simulink model "Par8_11"  (R2018a)
settings: Solver=FixedStepAuto  StartTime=0.0  StopTime=50  FixedStep=0.01  RelTol=1e-3
settings Model: Creator=wangluo  LastModifiedBy=wangluo

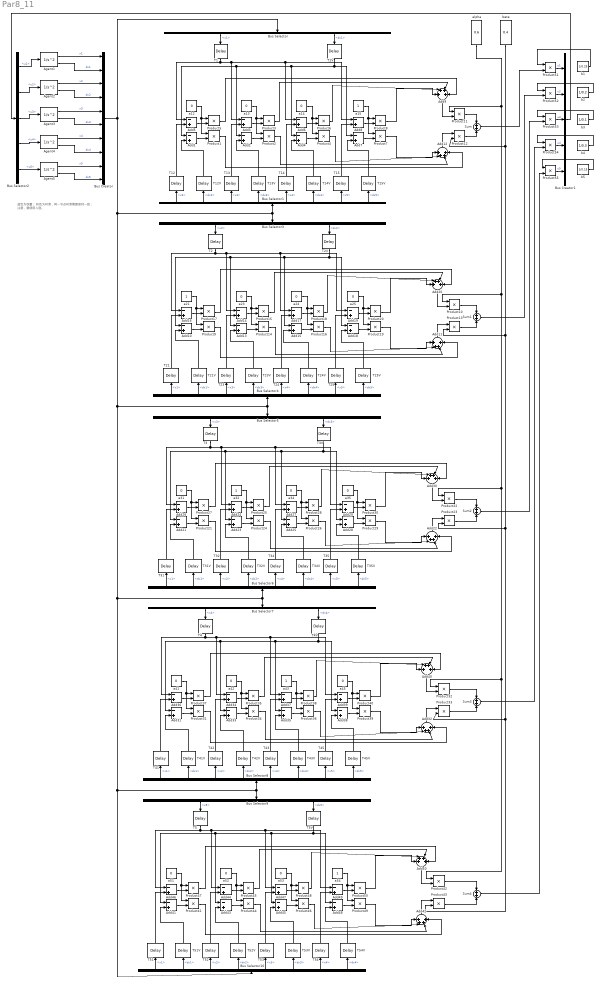
== system Par8_11 ==
  note: 蓝色为权重；
      | 粉色为时滞，同一节点时滞需要保持一致；
      | 注意，要使用入度。
  Add{1..8,10,13..19,21,23..29,31,33..39,41,43..49} (40 alike) : Sum  Inputs=-+
  Add{9,11..12,20,22,30,32,40,42,50} (10 alike) : Sum  Inputs=++++
  Agent1 : SecondOrderIntegrator  ICX=40  ICDXDT=4
  Agent2 : SecondOrderIntegrator  ICX=55  ICDXDT=5
  Agent3 : SecondOrderIntegrator  ICX=75  ICDXDT=20
  Agent4 : SecondOrderIntegrator  ICX=60  ICDXDT=10
  Agent5 : SecondOrderIntegrator  ICX=80  ICDXDT=20
  Bus Creator : BusCreator  Inputs=10
  Bus Creator1 : BusCreator  Inputs=5
  Bus Selector : BusSelector  OutputSignals=x1,dx1
  Bus Selector1 : BusSelector  OutputSignals=x2,dx2,x3,dx3,x4,dx4,x5,dx5
  Bus Selector10 : BusSelector  OutputSignals=x1,dx1,x2,dx2,x3,dx3,x4,dx4
  Bus Selector2 : BusSelector  OutputSignals=u1,u2,u3,u4,u5
  Bus Selector3 : BusSelector  OutputSignals=x2,dx2
  Bus Selector4 : BusSelector  OutputSignals=x1,dx1,x3,dx3,x4,dx4,x5,dx5
  Bus Selector5 : BusSelector  OutputSignals=x3,dx3
  Bus Selector6 : BusSelector  OutputSignals=x1,dx1,x2,dx2,x4,dx4,x5,dx5
  Bus Selector7 : BusSelector  OutputSignals=x4,dx4
  Bus Selector8 : BusSelector  OutputSignals=x1,dx1,x2,dx2,x3,dx3,x5,dx5
  Bus Selector9 : BusSelector  OutputSignals=x5,dx5
  Product{1..55} (55 alike) : Product
  Sum{,1..4} (5 alike) : Sum
  T{1..5,12..15,21,23..25,31..32,34..35,41..43,45,51..54} (25 alike) : TransportDelay  DelayTime=0
  T12V : TransportDelay  DelayTime=0
  T13V : TransportDelay  DelayTime=0
  T14V : TransportDelay  DelayTime=0
  T15V : TransportDelay  DelayTime=0
  T1V : TransportDelay  DelayTime=0
  T21V : TransportDelay  DelayTime=0
  T23V : TransportDelay  DelayTime=0
  T24V : TransportDelay  DelayTime=0
  T25V : TransportDelay  DelayTime=0
  T2V : TransportDelay  DelayTime=0
  T31V : TransportDelay  DelayTime=0
  T32V : TransportDelay  DelayTime=0
  T34V : TransportDelay  DelayTime=0
  T35V : TransportDelay  DelayTime=0
  T3V : TransportDelay  DelayTime=0
  T41V : TransportDelay  DelayTime=0
  T42V : TransportDelay  DelayTime=0
  T43V : TransportDelay  DelayTime=0
  T45V : TransportDelay  DelayTime=0
  T4V : TransportDelay  DelayTime=0
  T51V : TransportDelay  DelayTime=0
  T52V : TransportDelay  DelayTime=0
  T53V : TransportDelay  DelayTime=0
  T54V : TransportDelay  DelayTime=0
  T5V : TransportDelay  DelayTime=0
  a{12..14,23..25,31,34..35,41..42,45,51..53} (15 alike) : Constant  Value=0
  a{15,21,32,43,54} (5 alike) : Constant
  alpha : Constant  Value=0.6
  b1 : Constant  Value=1/0.25
  b2 : Constant  Value=1/0.2
  b3 : Constant  Value=1/0.1
  b4 : Constant  Value=1/0.3
  b5 : Constant  Value=1/0.15
  beta : Constant  Value=0.4
  wires:
  Agent1/1 -> Bus Creator/1  "x1"
  Agent1/2 -> Bus Creator/2  "dx1"
  Agent2/1 -> Bus Creator/3  "x2"
  Agent2/2 -> Bus Creator/4  "dx2"
  Agent3/1 -> Bus Creator/5  "x3"
  Agent3/2 -> Bus Creator/6  "dx3"
  Agent4/1 -> Bus Creator/7  "x4"
  Agent4/2 -> Bus Creator/8  "dx4"
  Agent5/1 -> Bus Creator/9  "x5"
  Agent5/2 -> Bus Creator/10  "dx5"
  Add5/1 -> Product5/2
  Add1/1 -> Product1/2
  a12/1 -> Product5/1, Product1/1
  Bus Selector1/1 -> T12/1  "<x2>"
  Bus Selector1/2 -> T12V/1  "<dx2>"
  a13/1 -> Product3/1, Product2/1
  Add3/1 -> Product3/2
  Add2/1 -> Product2/2
  a14/1 -> Product6/1, Product4/1
  Add6/1 -> Product6/2
  Add4/1 -> Product4/2
  a15/1 -> Product8/1, Product7/1
  Add8/1 -> Product8/2
  Add7/1 -> Product7/2
  Bus Selector1/4 -> T13V/1  "<dx3>"
  Bus Selector1/3 -> T13/1  "<x3>"
  Bus Selector1/6 -> T14V/1  "<dx4>"
  Bus Selector1/5 -> T14/1  "<x4>"
  Bus Selector1/8 -> T15V/1  "<dx5>"
  Bus Selector1/7 -> T15/1  "<x5>"
  Bus Selector/1 -> T1/1  "<x1>"
  Bus Selector/2 -> T1V/1  "<dx1>"
  Product11/1 -> Sum/1
  Product12/1 -> Sum/2
  Product7/1 -> Add12/1
  Product4/1 -> Add12/2
  Product2/1 -> Add12/3
  Product1/1 -> Add12/4
  Product8/1 -> Add9/1
  Product6/1 -> Add9/2
  Product3/1 -> Add9/3
  Product5/1 -> Add9/4
  Add12/1 -> Product12/1
  Add9/1 -> Product11/2
  Bus Selector2/1 -> Agent1/1  "<u1>"
  Sum/1 -> Product51/2
  Sum1/1 -> Product52/2
  Sum2/1 -> Product53/2
  Sum3/1 -> Product54/2
  Sum4/1 -> Product55/2
  Bus Selector2/2 -> Agent2/1  "<u2>"
  Bus Selector2/3 -> Agent3/1  "<u3>"
  Bus Selector2/4 -> Agent4/1  "<u4>"
  Bus Selector2/5 -> Agent5/1  "<u5>"
  Bus Selector4/3 -> T23/1  "<x3>"
  Bus Selector4/1 -> T21/1  "<x1>"
  Add20/1 -> Product10/2
  Product10/1 -> Sum1/1
  Product17/1 -> Add20/4
  a21/1 -> Product17/1, Product9/1
  Product15/1 -> Add20/3
  Add10/1 -> Product9/2
  Add13/1 -> Product14/2
  a24/1 -> Product18/1, Product16/1
  Bus Selector4/8 -> T25V/1  "<dx5>"
  Bus Selector4/7 -> T25/1  "<x5>"
  Product9/1 -> Add11/4
  Add19/1 -> Product20/2
  Product13/1 -> Sum1/2
  Add15/1 -> Product16/2
  Bus Selector4/6 -> T24V/1  "<dx4>"
  Product16/1 -> Add11/2
  Add17/1 -> Product18/2
  Bus Selector3/1 -> T2/1  "<x2>"
  Bus Selector4/5 -> T24/1  "<x4>"
  Bus Selector4/4 -> T23V/1  "<dx3>"
  Product19/1 -> Add11/1
  Add18/1 -> Product19/2
  a23/1 -> Product15/1, Product14/1
  a25/1 -> Product20/1, Product19/1
  Product14/1 -> Add11/3
  Product20/1 -> Add20/1
  Bus Selector3/2 -> T2V/1  "<dx2>"
  Product18/1 -> Add20/2
  Add11/1 -> Product13/1
  Add14/1 -> Product15/2
  Bus Selector4/2 -> T21V/1  "<dx1>"
  Add16/1 -> Product17/2
  Add30/1 -> Product22/2
  Product22/1 -> Sum2/1
  Product27/1 -> Add30/4
  a31/1 -> Product27/1, Product21/1
  Product25/1 -> Add30/3
  Add21/1 -> Product21/2
  Add23/1 -> Product24/2
  a34/1 -> Product28/1, Product26/1
  Bus Selector6/8 -> T35V/1  "<dx5>"
  Bus Selector6/7 -> T35/1  "<x5>"
  Product21/1 -> Add22/4
  Add29/1 -> Product30/2
  Product23/1 -> Sum2/2
  Add25/1 -> Product26/2
  Bus Selector6/6 -> T34V/1  "<dx4>"
  Product26/1 -> Add22/2
  Add27/1 -> Product28/2
  Bus Selector5/1 -> T3/1  "<x3>"
  Bus Selector6/5 -> T34/1  "<x4>"
  Product29/1 -> Add22/1
  Add28/1 -> Product29/2
  a32/1 -> Product25/1, Product24/1
  a35/1 -> Product30/1, Product29/1
  Product24/1 -> Add22/3
  Product30/1 -> Add30/1
  Bus Selector5/2 -> T3V/1  "<dx3>"
  Product28/1 -> Add30/2
  Add22/1 -> Product23/1
  Add24/1 -> Product25/2
  Add26/1 -> Product27/2
  Add40/1 -> Product32/2
  Product32/1 -> Sum3/1
  Product37/1 -> Add40/4
  a41/1 -> Product37/1, Product31/1
  Product35/1 -> Add40/3
  Add31/1 -> Product31/2
  Add33/1 -> Product34/2
  a43/1 -> Product38/1, Product36/1
  Product31/1 -> Add32/4
  Add39/1 -> Product40/2
  Product33/1 -> Sum3/2
  Add35/1 -> Product36/2
  Product36/1 -> Add32/2
  Add37/1 -> Product38/2
  Bus Selector7/1 -> T4/1  "<x4>"
  Product39/1 -> Add32/1
  Add38/1 -> Product39/2
  a42/1 -> Product35/1, Product34/1
  a45/1 -> Product40/1, Product39/1
  Product34/1 -> Add32/3
  Product40/1 -> Add40/1
  Bus Selector7/2 -> T4V/1  "<dx4>"
  Product38/1 -> Add40/2
  Add32/1 -> Product33/1
  Add34/1 -> Product35/2
  Add36/1 -> Product37/2
  Add50/1 -> Product42/2
  Product42/1 -> Sum4/1
  Product47/1 -> Add50/4
  alpha/1 -> Product11/1, Product42/1, Product32/1, Product22/1, Product10/1
  a51/1 -> Product47/1, Product41/1
  Product45/1 -> Add50/3
  Add41/1 -> Product41/2
  Add43/1 -> Product44/2
  a53/1 -> Product48/1, Product46/1
  beta/1 -> Product43/2, Product33/2, Product23/2, Product13/2, Product12/2
  Product41/1 -> Add42/4
  Add49/1 -> Product50/2
  Bus Creator/1 -> Bus Selector10/1, Bus Selector9/1, Bus Selector8/1, Bus Selector7/1, Bus Selector6/1, Bus Selector5/1, Bus Selector4/1, Bus Selector3/1, Bus Selector1/1, Bus Selector/1
  Product43/1 -> Sum4/2
  Add45/1 -> Product46/2
  Product46/1 -> Add42/2
  Add47/1 -> Product48/2
  Bus Selector9/1 -> T5/1  "<x5>"
  Product49/1 -> Add42/1
  Add48/1 -> Product49/2
  a52/1 -> Product45/1, Product44/1
  a54/1 -> Product50/1, Product49/1
  Product44/1 -> Add42/3
  Product50/1 -> Add50/1
  Bus Selector9/2 -> T5V/1  "<dx5>"
  Product48/1 -> Add50/2
  Add42/1 -> Product43/1
  Add44/1 -> Product45/2
  Add46/1 -> Product47/2
  Bus Selector6/4 -> T32V/1  "<dx2>"
  Bus Selector6/3 -> T32/1  "<x2>"
  Bus Selector6/2 -> T31V/1  "<dx1>"
  Bus Selector6/1 -> T31/1  "<x1>"
  Bus Selector8/1 -> T41/1  "<x1>"
  Bus Selector8/2 -> T41V/1  "<dx1>"
  Bus Selector8/3 -> T42/1  "<x2>"
  Bus Selector8/4 -> T42V/1  "<dx2>"
  Bus Selector8/5 -> T43/1  "<x3>"
  Bus Selector8/6 -> T43V/1  "<dx3>"
  Bus Selector8/7 -> T45/1  "<x5>"
  Bus Selector8/8 -> T45V/1  "<dx5>"
  Bus Selector10/1 -> T51/1  "<x1>"
  Bus Selector10/2 -> T51V/1  "<dx1>"
  Bus Selector10/3 -> T52/1  "<x2>"
  Bus Selector10/4 -> T52V/1  "<dx2>"
  Bus Selector10/5 -> T53/1  "<x3>"
  Bus Selector10/6 -> T53V/1  "<dx3>"
  Bus Selector10/7 -> T54/1  "<x4>"
  Bus Selector10/8 -> T54V/1  "<dx4>"
  T21/1 -> Add16/2
  T21V/1 -> Add10/2
  T1/1 -> Add3/1, Add6/1, Add8/1, Add5/1
  T1V/1 -> Add7/1, Add4/1, Add2/1, Add1/1
  T12/1 -> Add5/2
  T13V/1 -> Add2/2
  T12V/1 -> Add1/2
  T13/1 -> Add3/2
  T14/1 -> Add6/2
  T14V/1 -> Add4/2
  T15/1 -> Add8/2
  T15V/1 -> Add7/2
  T2/1 -> Add16/1, Add14/1, Add17/1, Add19/1
  T25V/1 -> Add18/2
  T25/1 -> Add19/2
  T24V/1 -> Add15/2
  T24/1 -> Add17/2
  T23V/1 -> Add13/2
  T23/1 -> Add14/2
  T2V/1 -> Add18/1, Add15/1, Add13/1, Add10/1
  T3/1 -> Add26/1, Add24/1, Add29/1, Add27/1
  T3V/1 -> Add28/1, Add25/1, Add23/1, Add21/1
  T35V/1 -> Add28/2
  T35/1 -> Add29/2
  T34V/1 -> Add25/2
  T34/1 -> Add27/2
  T32V/1 -> Add23/2
  T32/1 -> Add24/2
  T31/1 -> Add26/2
  T31V/1 -> Add21/2
  T4V/1 -> Add38/1, Add35/1, Add31/1, Add33/1
  T4/1 -> Add36/1, Add34/1, Add37/1, Add39/1
  T45V/1 -> Add38/2
  T45/1 -> Add39/2
  T43V/1 -> Add35/2
  T43/1 -> Add37/2
  T42V/1 -> Add33/2
  T42/1 -> Add34/2
  T41V/1 -> Add31/2
  T41/1 -> Add36/2
  T5V/1 -> Add48/1, Add45/1, Add41/1, Add43/1
  T5/1 -> Add46/1, Add44/1, Add47/1, Add49/1
  T51/1 -> Add46/2
  T54V/1 -> Add48/2
  T51V/1 -> Add41/2
  T52/1 -> Add44/2
  T52V/1 -> Add43/2
  T53/1 -> Add47/2
  T53V/1 -> Add45/2
  T54/1 -> Add49/2
  b2/1 -> Product52/1
  Product52/1 -> Bus Creator1/2  "u2"
  Product55/1 -> Bus Creator1/5  "u5"
  Product51/1 -> Bus Creator1/1  "u1"
  Product53/1 -> Bus Creator1/3  "u3"
  Product54/1 -> Bus Creator1/4  "u4"
  b3/1 -> Product53/1
  b1/1 -> Product51/1
  b4/1 -> Product54/1
  b5/1 -> Product55/1
  Bus Creator1/1 -> Bus Selector2/1
